simulink model "nmsRR"  (R2021a)
settings: Solver=ode15s  StartTime=0.0  StopTime=t  MaxStep=1e-2  RelTol=1e-2
StartFcn:
  | tic
StopFcn:
  | toc
  | 
  | 
  | %if GimbalLockFlag
  |  % fprintf(2, 'Almost reached Gimbal Lock of IMU. Simulation stopped.\n')
  | %end
  | 
  | %fprintf('Elapsed time: %4.2f sec (%4.2f%% realtime)\n', a, tout(end)/a*100)
undefined symbols (not defined in the file): Balance02, Balance13, BalanceTrunk, BasisStim, CompensateSwing, CompliantLeg, FlexAnkle, Ground, ICs, init_des_left, init_des_right, init_l_left, init_l_right, init_q_del, init_sensor_body, init_sensor_world, init_v_left, init_v_right, LateralControl, mParams, PreventKneeOverextension, StepDur, Target02, Target13, theta0, X, Y, Z
libraries: simulink_extras x133, nesl_utility x105, sm_lib x88, simulink x72, robotcorelib x5, dspinverses x5, dspswit3 x2, vrlib x2, robotmaniplib x1
(part 4 of 8)

== system nmsRR/Body and Contact Model/L Leg/Thigh ==
  Solid : sm_lib/Body Elements/Brick Solid  Commented=on  GraphicAmbientColor=[0.15 0.15 0.15 1.0]  BasedOnType=Density  BrickDimensions="[mParams.bodies.thigh.d  mParams.bodies.thigh.l*(1-mParams.bodies.thigh.ThPos)   mParams.bodies.thigh.b]"  BrickDimensionUnits=m  CenterOfMass=-mParams.bodies.thigh.CG*(1-mParams.bodies.thigh.ThPos)  CenterOfMassUnits=m  GraphicDiffuseColor=[1 0.5 0.5]  Density=2.7  DensityUnits=g/cm^3  DoExposeReferenceFrame=on  GraphicEmissiveColor=[0 0 0 1.0]  ExportEntireGeometry=off  SerializedFrames=<Frames/>  MarkerShape=Sphere  MarkerSize=10  GraphicType=FromGeometry  InertiaType=Custom  Mass=mParams.bodies.thigh.m*(1-mParams.bodies.thigh.ThPos)  MassUnits=kg  MomentsOfInertia=mParams.bodies.thigh.In*[(1-mParams.bodies.thigh.ThPos); (1-mParams.bodies.thigh.ThPos)^3; (1-mParams.bodies.thigh.ThPos)^3]  MomentsOfInertiaUnits=kg*m^2  GraphicOpacity=1.0  ProductsOfInertia=[0 0 0]  ProductsOfInertiaUnits=kg*m^2  GraphicShininess=75  GraphicSpecularColor=[0.5 0.5 0.5 1.0]  GraphicVisPropType=SimpleVisualProperties
  Solid1 : sm_lib/Body Elements/Brick Solid  GraphicAmbientColor=[0.15 0.15 0.15 1.0]  BasedOnType=Density  BrickDimensions=[mParams.bodies.thigh.d mParams.bodies.thigh.l mParams.bodies.thigh.b]  BrickDimensionUnits=m  CenterOfMass=mParams.bodies.thigh.CG  CenterOfMassUnits=m  GraphicDiffuseColor=[1 0.5 0.5]  Density=2.7  DensityUnits=g/cm^3  DoExposeReferenceFrame=on  GraphicEmissiveColor=[0 0 0 1.0]  ExportEntireGeometry=off  SerializedFrames=<Frames><Frame><Id>Frame1</Id><Value><Name>F1</Name><Origin><Source>CenterOfMassFrame</Source><FeatureName></FeatureName></Origin><PrimaryAxis><DefinedDirection>+Z</DefinedDirection><Source>ReferenceFrame</Source><SourceDirection>+Z</SourceDirection><FeatureName></FeatureName></PrimaryAxis><SecondaryAxis><DefinedDirection>+X</DefinedDirection><Source>ReferenceFrame</Source><SourceDirection>+X</SourceDirection><FeatureName></FeatureName></SecondaryAxis></Value></Frame></Frames>  MarkerShape=Sphere  MarkerSize=10  GraphicType=FromGeometry  InertiaType=Custom  Mass=mParams.bodies.thigh.m  MassUnits=kg  MomentsOfInertia=mParams.bodies.thigh.In  MomentsOfInertiaUnits=kg*m^2  GraphicOpacity=1.0  ProductsOfInertia=[0 0 0]  ProductsOfInertiaUnits=kg*m^2  GraphicShininess=75  GraphicSpecularColor=[0.5 0.5 0.5 1.0]  GraphicVisPropType=SimpleVisualProperties
  Transform CG to MidSegment : sm_lib/Frames and Transforms/Rigid Transform  TranslationMethod=Cartesian  TranslationStandardOffset=0  TranslationLengthUnit=m  TranslationStandardAxis=+Y  TranslationCartesianOffset=[0 -mParams.bodies.thigh.l/2 0]  TranslationROffset=0  TranslationROffsetUnits=m  TranslationZOffset=0  TranslationZOffsetUnits=m  TranslationThetaOffset=0  TranslationThetaOffsetUnits=deg  RotationMethod=None  RotationAngleUnits=deg  RotationStandardAxis=+X  RotationAngle=90  RotationArbitraryAxis=[0 0 1]  FollAlignAxisA=+X  BaseAlignAxisA=+Y  FollAlignAxisB=+Y  BaseAlignAxisB=+Z  RotationSequenceAxes=FollowerAxes  RotationSequence=XYX  RotationSequenceAngles=[0 0 0]  RotationSequenceAnglesUnits=deg  RotationMatrix=[1 0 0; 0 1 0; 0 0 1]
  Transform CS1 to MidSegment : sm_lib/Frames and Transforms/Rigid Transform  TranslationMethod=Cartesian  TranslationStandardOffset=0  TranslationLengthUnit=m  TranslationStandardAxis=+Y  TranslationCartesianOffset=[0 -mParams.bodies.thigh.l/2 0]  TranslationROffset=0  TranslationROffsetUnits=m  TranslationZOffset=0  TranslationZOffsetUnits=m  TranslationThetaOffset=0  TranslationThetaOffsetUnits=deg  RotationMethod=None  RotationAngleUnits=deg  RotationStandardAxis=+X  RotationAngle=-90  RotationArbitraryAxis=[0 0 1]  FollAlignAxisA=+X  BaseAlignAxisA=+Y  FollAlignAxisB=+Y  BaseAlignAxisB=+Z  RotationSequenceAxes=FollowerAxes  RotationSequence=XYX  RotationSequenceAngles=[0 0 0]  RotationSequenceAnglesUnits=deg  RotationMatrix=[1 0 0; 0 1 0; 0 0 1]
  CS1 : PMIOPort  Side=Left
  CS2 : PMIOPort  Port=2  Side=Right
  connections:
  Transform CG to MidSegment/LConn1 -- Solid1/RConn1 -- Transform CS1 to MidSegment/RConn1
  Transform CS1 to MidSegment/LConn1 -- CS1/RConn1
  Transform CG to MidSegment/RConn1 -- CS2/RConn1

== system nmsRR/Body and Contact Model/Push in x-direction/ Timer Phase 1 ==
  R : Inport
  Clock1 : Clock
  Clock3 : Clock
      settings: Decimation=4
  NOT : Logic  Operator=NOT  AllPortsSameDT=off  OutDataTypeStr=boolean
  Resettable Subsystem : Subsystem  TreatAsAtomicUnit=on
  Sum1 : Sum  Inputs=|+-  InputSameDT=on  SaturateOnIntegerOverflow=on  OutDataTypeStr=Inherit: Same as first input
  Switch2 : Switch  Criteria=u2 > Threshold  RndMeth=Zero  ZeroCross=off
  Out : Outport  VectorParamsAs1DForOutWhenUnconnected=off
  wires:
  Clock1/1 -> Sum1/1
  Clock3/1 -> Switch2/3, Resettable Subsystem/1(In1)
  Sum1/1 -> Out/1
  R/1 -> NOT/1, Switch2/2
  Switch2/1 -> Sum1/2
  Resettable Subsystem/1(Out1) -> Switch2/1
  NOT/1 -> Resettable Subsystem/Enable

== system nmsRR/Body and Contact Model/Push in y-direction/ Timer Phase 1 ==
  R : Inport
  Clock1 : Clock
  Clock3 : Clock
      settings: Decimation=4
  NOT : Logic  Operator=NOT  AllPortsSameDT=off  OutDataTypeStr=boolean
  Resettable Subsystem : Subsystem  TreatAsAtomicUnit=on
  Sum1 : Sum  Inputs=|+-  InputSameDT=on  SaturateOnIntegerOverflow=on  OutDataTypeStr=Inherit: Same as first input
  Switch2 : Switch  Criteria=u2 > Threshold  RndMeth=Zero  ZeroCross=off
  Out : Outport  VectorParamsAs1DForOutWhenUnconnected=off
  wires:
  Clock1/1 -> Sum1/1
  Clock3/1 -> Switch2/3, Resettable Subsystem/1(In1)
  Sum1/1 -> Out/1
  R/1 -> NOT/1, Switch2/2
  Switch2/1 -> Sum1/2
  Resettable Subsystem/1(Out1) -> Switch2/1
  NOT/1 -> Resettable Subsystem/Enable

== system nmsRR/Body and Contact Model/R Leg/Ankle Mechanical Limits ==
  note: Overflexion Torque
  note: Joint Limits
  note: Overextension Torque
  dq [rad/s] : Inport
  q [rad] : Inport  Port=2
  Gain1 : Gain  Gain=mParams.joints.ankle.kStop
  Gain2 : Gain  Gain=-1
  Gain3 : Gain  Gain=mParams.joints.ankle.kStop
  Gain4 : Gain  Gain=1/mParams.joints.ankle.wMaxStop
  Gain5 : Gain  Gain=-1
  Gain6 : Gain  Gain=-1
  Limit Knee Range : simulink/Logic and Bit Operations/Interval Test  Commented=on  IntervalClosedRight=on  uplimit=mParams.joints.ankle.MaxPitch + 20*pi/180  IntervalClosedLeft=on  lowlimit=mParams.joints.ankle.MinPitch - 20*pi/180  OutDataTypeStr=boolean
      settings: AttributesFormatString=|
      | Lower limits: %<lowlimit>
      | Upper limits: %<uplimit>
  Logical Operator3 : Logic  Commented=on  Operator=NOT  AllPortsSameDT=off  OutDataTypeStr=boolean
  Product1 : Product  Inputs=4
  Product2 : Product  Inputs=4
  Stop Simulation1 : Stop  Commented=on
  Sum : Sum  Inputs=|+-
  Sum1 : Sum  Inputs=|+-
  Sum2 : Sum
  Sum3 : Sum  Inputs=|-+
  Sum4 : Sum  Inputs=|-+
  above upper limit? : simulink/Logic and Bit Operations/Compare To Zero  relop=>  OutDataTypeStr=boolean  ZeroCross=off
  below lower limit? : simulink/Logic and Bit Operations/Compare To Zero  relop=<  OutDataTypeStr=boolean  ZeroCross=off
  const : Constant
  const1 : Constant
  mech limit pushes back? : simulink/Logic and Bit Operations/Compare To Zero  relop=>  OutDataTypeStr=boolean  ZeroCross=off
  mech limit pushes back?. : simulink/Logic and Bit Operations/Compare To Zero  relop=>  OutDataTypeStr=boolean  ZeroCross=off
  overextension angle : Constant  Value=mParams.joints.ankle.MaxPitch
  overflexion angle : Constant  Value=mParams.joints.ankle.MinPitch
  tau [Nm] : Outport  VectorParamsAs1DForOutWhenUnconnected=off
  wires:
  Gain5/1 -> Sum2/2
  Gain4/1 -> Gain2/1, Sum4/1
  const1/1 -> Sum4/2
  Sum4/1 -> Product2/3, mech limit pushes back?./1
  Gain1/1 -> Product2/2, below lower limit?/1
  mech limit pushes back?./1 -> Product2/4
  below lower limit?/1 -> Product2/1
  Product2/1 -> Gain5/1
  Product1/1 -> Gain6/1
  above upper limit?/1 -> Product1/1
  mech limit pushes back?/1 -> Product1/4
  Gain3/1 -> above upper limit?/1, Product1/2
  Sum3/1 -> mech limit pushes back?/1, Product1/3
  const/1 -> Sum3/2
  dq [rad/s]/1 -> Gain4/1
  overextension angle/1 -> Sum/2
  q [rad]/1 -> Sum/1, Limit Knee Range/1, Sum1/1
  Sum/1 -> Gain3/1
  Sum1/1 -> Gain1/1
  overflexion angle/1 -> Sum1/2
  Sum2/1 -> tau [Nm]/1
  Gain2/1 -> Sum3/1
  Gain6/1 -> Sum2/1
  Limit Knee Range/1 -> Logical Operator3/1
  Logical Operator3/1 -> Stop Simulation1/1

== system nmsRR/Body and Contact Model/R Leg/Foot1 ==
  "  XYZ Sensor " : Subsystem
  "  XYZ Sensor Ball left" : Subsystem
  B Transform : sm_lib/Frames and Transforms/Rigid Transform  TranslationMethod=Cartesian  TranslationStandardOffset=0  TranslationLengthUnit=m  TranslationStandardAxis=+Y  TranslationCartesianOffset=[ mParams.bodies.foot.compensation mParams.bodies.foot.l/2 0]  TranslationROffset=0  TranslationROffsetUnits=m  TranslationZOffset=0  TranslationZOffsetUnits=m  TranslationThetaOffset=0  TranslationThetaOffsetUnits=deg  RotationMethod=None  RotationAngleUnits=deg  RotationStandardAxis=+X  RotationAngle=90  RotationArbitraryAxis=[0 0 1]  FollAlignAxisA=+X  BaseAlignAxisA=+Y  FollAlignAxisB=+Y  BaseAlignAxisB=+Z  RotationSequenceAxes=FollowerAxes  RotationSequence=XYX  RotationSequenceAngles=[0 0 0]  RotationSequenceAnglesUnits=deg  RotationMatrix=[1 0 0; 0 1 0; 0 0 1]
  LB Transform : sm_lib/Frames and Transforms/Rigid Transform  TranslationMethod=Cartesian  TranslationStandardOffset=0  TranslationLengthUnit=m  TranslationStandardAxis=+Y  TranslationCartesianOffset="[mParams.bodies.foot.l/2 -mParams.bodies.foot.compensation  -mParams.bodies.foot.BallWidth/2]"  TranslationROffset=0  TranslationROffsetUnits=m  TranslationZOffset=0  TranslationZOffsetUnits=m  TranslationThetaOffset=0  TranslationThetaOffsetUnits=deg  RotationMethod=None  RotationAngleUnits=deg  RotationStandardAxis=+X  RotationAngle=90  RotationArbitraryAxis=[0 0 1]  FollAlignAxisA=+X  BaseAlignAxisA=+Y  FollAlignAxisB=+Y  BaseAlignAxisB=+Z  RotationSequenceAxes=FollowerAxes  RotationSequence=XYX  RotationSequenceAngles=[0 0 0]  RotationSequenceAnglesUnits=deg  RotationMatrix=[1 0 0; 0 1 0; 0 0 1]
  LH Transform : sm_lib/Frames and Transforms/Rigid Transform  TranslationMethod=Cartesian  TranslationStandardOffset=0  TranslationLengthUnit=m  TranslationStandardAxis=+Y  TranslationCartesianOffset="[-mParams.bodies.foot.l/2 -mParams.bodies.foot.compensation  -mParams.bodies.foot.HeelWidth/2]"  TranslationROffset=0  TranslationROffsetUnits=m  TranslationZOffset=0  TranslationZOffsetUnits=m  TranslationThetaOffset=0  TranslationThetaOffsetUnits=deg  RotationMethod=None  RotationAngleUnits=deg  RotationStandardAxis=+X  RotationAngle=90  RotationArbitraryAxis=[0 0 1]  FollAlignAxisA=+X  BaseAlignAxisA=+Y  FollAlignAxisB=+Y  BaseAlignAxisB=+Z  RotationSequenceAxes=FollowerAxes  RotationSequence=XYX  RotationSequenceAngles=[0 0 0]  RotationSequenceAnglesUnits=deg  RotationMatrix=[1 0 0; 0 1 0; 0 0 1]
  RB Transform : sm_lib/Frames and Transforms/Rigid Transform  TranslationMethod=Cartesian  TranslationStandardOffset=0  TranslationLengthUnit=m  TranslationStandardAxis=+Z  TranslationCartesianOffset="[mParams.bodies.foot.l/2 -mParams.bodies.foot.compensation  mParams.bodies.foot.BallWidth/2]"  TranslationROffset=0  TranslationROffsetUnits=m  TranslationZOffset=0  TranslationZOffsetUnits=m  TranslationThetaOffset=0  TranslationThetaOffsetUnits=deg  RotationMethod=None  RotationAngleUnits=deg  RotationStandardAxis=+Z  RotationAngle=0.0  RotationArbitraryAxis=[0 0 1]  FollAlignAxisA=+X  BaseAlignAxisA=+Y  FollAlignAxisB=+Y  BaseAlignAxisB=+Z  RotationSequenceAxes=FollowerAxes  RotationSequence=XYX  RotationSequenceAngles=[0 0 0]  RotationSequenceAnglesUnits=deg  RotationMatrix=[1 0 0; 0 1 0; 0 0 1]
  RH Transform : sm_lib/Frames and Transforms/Rigid Transform  TranslationMethod=Cartesian  TranslationStandardOffset=0  TranslationLengthUnit=m  TranslationStandardAxis=+Z  TranslationCartesianOffset="[-mParams.bodies.foot.l/2 -mParams.bodies.foot.compensation  mParams.bodies.foot.HeelWidth/2]"  TranslationROffset=0  TranslationROffsetUnits=m  TranslationZOffset=0  TranslationZOffsetUnits=m  TranslationThetaOffset=0  TranslationThetaOffsetUnits=deg  RotationMethod=None  RotationAngleUnits=deg  RotationStandardAxis=+Z  RotationAngle=0.0  RotationArbitraryAxis=[0 0 1]  FollAlignAxisA=+X  BaseAlignAxisA=+Y  FollAlignAxisB=+Y  BaseAlignAxisB=+Z  RotationSequenceAxes=FollowerAxes  RotationSequence=XYX  RotationSequenceAngles=[0 0 0]  RotationSequenceAnglesUnits=deg  RotationMatrix=[1 0 0; 0 1 0; 0 0 1]
  Solid1 : sm_lib/Body Elements/Brick Solid  GraphicAmbientColor=[0.15 0.15 0.15 1.0]  BasedOnType=Density  BrickDimensions="[mParams.bodies.foot.l  mParams.bodies.foot.d mParams.bodies.foot.b]"  BrickDimensionUnits=m  CenterOfMass=mParams.bodies.foot.CG  CenterOfMassUnits=m  GraphicDiffuseColor=[1 0.5 0.5]  Density=2.7  DensityUnits=g/cm^3  DoExposeReferenceFrame=on  GraphicEmissiveColor=[0 0 0 1.0]  ExportEntireGeometry=off  SerializedFrames=<Frames><Frame><Id>Frame1</Id><Value><Name>CG</Name><Origin><Source>CenterOfMassFrame</Source><FeatureName></FeatureName></Origin><PrimaryAxis><DefinedDirection>+Z</DefinedDirection><Source>ReferenceFrame</Source><SourceDirection>+Z</SourceDirection><FeatureName></FeatureName></PrimaryAxis><SecondaryAxis><DefinedDirection>+X</DefinedDirection><Source>ReferenceFrame</Source><SourceDirection>+X</SourceDirection><FeatureName></FeatureName></SecondaryAxis></Value></Frame></Frames>  MarkerShape=Sphere  MarkerSize=10  GraphicType=FromGeometry  InertiaType=Custom  Mass=mParams.bodies.foot.m  MassUnits=kg  MomentsOfInertia=mParams.bodies.foot.In  MomentsOfInertiaUnits=kg*m^2  GraphicOpacity=1.0  ProductsOfInertia=[0 0 0]  ProductsOfInertiaUnits=kg*m^2  GraphicShininess=75  GraphicSpecularColor=[0.5 0.5 0.5 1.0]  GraphicVisPropType=SimpleVisualProperties
  Terminator : Terminator
  Terminator1 : Terminator
  To Workspace4 : ToWorkspace  VariableName=Ball_right  SampleTime=-1
      settings: Save2DSignal=2-D array (concatenate along first dimension)
  Transform Ankle to MidSegment : sm_lib/Frames and Transforms/Rigid Transform  TranslationMethod=Cartesian  TranslationStandardOffset=0  TranslationLengthUnit=m  TranslationStandardAxis=+Y  TranslationCartesianOffset=mParams.bodies.foot.AnkleToMid  TranslationROffset=0  TranslationROffsetUnits=m  TranslationZOffset=0  TranslationZOffsetUnits=m  TranslationThetaOffset=0  TranslationThetaOffsetUnits=deg  RotationMethod=RotationSequence  RotationAngleUnits=deg  RotationStandardAxis=+X  RotationAngle=-90  RotationArbitraryAxis=[0 0 1]  FollAlignAxisA=+X  BaseAlignAxisA=+Y  FollAlignAxisB=+Y  BaseAlignAxisB=+Z  RotationSequenceAxes=FollowerAxes  RotationSequence=ZXY  RotationSequenceAngles=[90 0 0]  RotationSequenceAnglesUnits=deg  RotationMatrix=[1 0 0; 0 1 0; 0 0 1]
  CS1 : PMIOPort  Side=Left
  Left Ball : PMIOPort  Port=2  Side=Right
  Left Heel : PMIOPort  Port=3  Side=Left
  Right Ball : PMIOPort  Port=4  Side=Right
  Right Heel : PMIOPort  Port=5  Side=Left
  Out1 : Outport  VectorParamsAs1DForOutWhenUnconnected=off
  tag scope: Ball_right=global
  wires:
  "  XYZ Sensor "/1(p_bLH [m x3]) -> Out1/1
  "  XYZ Sensor Ball left"/2(v_bLH [m/s x3]) -> Terminator/1
  "  XYZ Sensor Ball left"/1(p_bLH [m x3]) -> To Workspace4/1, [Ball_right]
  "  XYZ Sensor "/2(v_bLH [m/s x3]) -> Terminator1/1
  connections:
  Transform Ankle to MidSegment/RConn1 -- B Transform/LConn1 -- RB Transform/LConn1 -- Solid1/RConn1 -- RH Transform/LConn1 -- LH Transform/LConn1 -- LB Transform/LConn1
  Transform Ankle to MidSegment/LConn1 -- CS1/RConn1
  Left Heel/RConn1 -- LH Transform/RConn1
  Left Ball/RConn1 -- LB Transform/RConn1
  Right Heel/RConn1 -- RH Transform/RConn1
  Right Ball/RConn1 -- RB Transform/RConn1
  Solid1/LConn1 -- "  XYZ Sensor "/LConn1
  B Transform/RConn1 -- "  XYZ Sensor Ball left"/LConn1

== system nmsRR/Body and Contact Model/R Leg/Hip Pitch Mechanical Limits ==
  note: Overextension Torque
  note: Joint Limits
  note: Overflexion Torque
  dq [rad/s] : Inport
  q [rad] : Inport  Port=2
  Gain1 : Gain  Gain=mParams.joints.hip.kStop
  Gain2 : Gain  Gain=-1
  Gain3 : Gain  Gain=mParams.joints.hip.kStop
  Gain4 : Gain  Gain=1/mParams.joints.hip.wMaxStop
  Gain5 : Gain  Gain=-1
  Gain6 : Gain  Gain=-1
  Limit Joint Range : simulink/Logic and Bit Operations/Interval Test  Commented=on  IntervalClosedRight=on  uplimit=mParams.joints.hip.MaxPitch + 20*pi/180  IntervalClosedLeft=on  lowlimit=mParams.joints.hip.MinPitch - 20*pi/180  OutDataTypeStr=boolean
      settings: AttributesFormatString=|
      | Lower limits: %<lowlimit>
      | Upper limits: %<uplimit>
  Logical Operator3 : Logic  Commented=on  Operator=NOT  AllPortsSameDT=off  OutDataTypeStr=boolean
  Product1 : Product  Inputs=4
  Product2 : Product  Inputs=4
  Stop Simulation1 : Stop  Commented=on
  Sum : Sum  Inputs=|+-
  Sum1 : Sum  Inputs=|+-
  Sum2 : Sum
  Sum3 : Sum  Inputs=|-+
  Sum4 : Sum  Inputs=|-+
  above upper limit? : simulink/Logic and Bit Operations/Compare To Zero  relop=>  OutDataTypeStr=boolean  ZeroCross=off
  below lower limit? : simulink/Logic and Bit Operations/Compare To Zero  relop=<  OutDataTypeStr=boolean  ZeroCross=off
  const : Constant
  const1 : Constant
  mech limit pushes back? : simulink/Logic and Bit Operations/Compare To Zero  relop=>  OutDataTypeStr=boolean  ZeroCross=off
  mech limit pushes back?. : simulink/Logic and Bit Operations/Compare To Zero  relop=>  OutDataTypeStr=boolean  ZeroCross=off
  overextension angle : Constant  Value=mParams.joints.hip.MaxPitch
  overflexion angle : Constant  Value=mParams.joints.hip.MinPitch
  tau [Nm] : Outport  VectorParamsAs1DForOutWhenUnconnected=off
  wires:
  Logical Operator3/1 -> Stop Simulation1/1
  Limit Joint Range/1 -> Logical Operator3/1
  Gain6/1 -> Sum2/1
  Gain2/1 -> Sum3/1
  Sum2/1 -> tau [Nm]/1
  overflexion angle/1 -> Sum1/2
  Sum1/1 -> Gain1/1
  Sum/1 -> Gain3/1
  q [rad]/1 -> Sum/1, Sum1/1, Limit Joint Range/1
  overextension angle/1 -> Sum/2
  dq [rad/s]/1 -> Gain4/1
  const/1 -> Sum3/2
  Sum3/1 -> Product1/3, mech limit pushes back?/1
  Gain3/1 -> Product1/2, above upper limit?/1
  mech limit pushes back?/1 -> Product1/4
  above upper limit?/1 -> Product1/1
  Product1/1 -> Gain6/1
  Product2/1 -> Gain5/1
  below lower limit?/1 -> Product2/1
  mech limit pushes back?./1 -> Product2/4
  Gain1/1 -> Product2/2, below lower limit?/1
  Sum4/1 -> mech limit pushes back?./1, Product2/3
  const1/1 -> Sum4/2
  Gain4/1 -> Sum4/1, Gain2/1
  Gain5/1 -> Sum2/2

== system nmsRR/Body and Contact Model/R Leg/Hip Roll Mechanical Limits ==
  note: Overextension Torque
  note: Joint Limits
  note: Overflexion Torque
  dq [rad/s] : Inport
  q [rad] : Inport  Port=2
  Gain1 : Gain  Gain=mParams.joints.hip.kStop
  Gain2 : Gain  Gain=-1
  Gain3 : Gain  Gain=mParams.joints.hip.kStop
  Gain4 : Gain  Gain=1/mParams.joints.hip.wMaxStop
  Gain5 : Gain  Gain=-1
  Gain6 : Gain  Gain=-1
  Limit Joint Range : simulink/Logic and Bit Operations/Interval Test  Commented=on  IntervalClosedRight=on  uplimit=mParams.joints.hip.MaxRoll + 20*pi/180  IntervalClosedLeft=on  lowlimit=mParams.joints.hip.MinRoll - 20*pi/180  OutDataTypeStr=boolean
      settings: AttributesFormatString=|
      | Lower limits: %<lowlimit>
      | Upper limits: %<uplimit>
  Logical Operator3 : Logic  Commented=on  Operator=NOT  AllPortsSameDT=off  OutDataTypeStr=boolean
  Product1 : Product  Inputs=4
  Product2 : Product  Inputs=4
  Stop Simulation1 : Stop  Commented=on
  Sum : Sum  Inputs=|+-
  Sum1 : Sum  Inputs=|+-
  Sum2 : Sum
  Sum3 : Sum  Inputs=|-+
  Sum4 : Sum  Inputs=|-+
  above upper limit? : simulink/Logic and Bit Operations/Compare To Zero  relop=>  OutDataTypeStr=boolean  ZeroCross=off
  below lower limit? : simulink/Logic and Bit Operations/Compare To Zero  relop=<  OutDataTypeStr=boolean  ZeroCross=off
  const : Constant
  const1 : Constant
  mech limit pushes back? : simulink/Logic and Bit Operations/Compare To Zero  relop=>  OutDataTypeStr=boolean  ZeroCross=off
  mech limit pushes back?. : simulink/Logic and Bit Operations/Compare To Zero  relop=>  OutDataTypeStr=boolean  ZeroCross=off
  overextension angle : Constant  Value=mParams.joints.hip.MaxRoll
  overflexion angle : Constant  Value=mParams.joints.hip.MinRoll
  tau [Nm] : Outport  VectorParamsAs1DForOutWhenUnconnected=off
  wires:
  Limit Joint Range/1 -> Logical Operator3/1
  Gain6/1 -> Sum2/1
  Gain2/1 -> Sum3/1
  Sum2/1 -> tau [Nm]/1
  overflexion angle/1 -> Sum1/2
  Sum1/1 -> Gain1/1
  Sum/1 -> Gain3/1
  q [rad]/1 -> Sum/1, Sum1/1, Limit Joint Range/1
  overextension angle/1 -> Sum/2
  dq [rad/s]/1 -> Gain4/1
  const/1 -> Sum3/2
  Sum3/1 -> Product1/3, mech limit pushes back?/1
  Gain3/1 -> Product1/2, above upper limit?/1
  mech limit pushes back?/1 -> Product1/4
  above upper limit?/1 -> Product1/1
  Product1/1 -> Gain6/1
  Product2/1 -> Gain5/1
  below lower limit?/1 -> Product2/1
  mech limit pushes back?./1 -> Product2/4
  Gain1/1 -> Product2/2, below lower limit?/1
  Sum4/1 -> mech limit pushes back?./1, Product2/3
  const1/1 -> Sum4/2
  Gain4/1 -> Sum4/1, Gain2/1
  Gain5/1 -> Sum2/2
  Logical Operator3/1 -> Stop Simulation1/1

== system nmsRR/Body and Contact Model/R Leg/Knee Mechanical Limits ==
  note: Overextension Torque
  note: Joint Limits
  note: Overflexion Torque
  dq [rad/s] : Inport
  q [rad] : Inport  Port=2
  Gain1 : Gain  Gain=mParams.joints.knee.kStop
  Gain2 : Gain  Gain=-1
  Gain3 : Gain  Gain=mParams.joints.knee.kStop
  Gain4 : Gain  Gain=1/mParams.joints.knee.wMaxStop
  Gain5 : Gain  Gain=-1
  Gain6 : Gain  Gain=-1
  Limit Knee Range : simulink/Logic and Bit Operations/Interval Test  IntervalClosedRight=on  uplimit=mParams.joints.knee.MaxPitch + 20*pi/180  IntervalClosedLeft=on  lowlimit=mParams.joints.knee.MinPitch - 20*pi/180  OutDataTypeStr=boolean
      settings: AttributesFormatString=|
      | Lower limits: %<lowlimit>
      | Upper limits: %<uplimit>
  Logical Operator3 : Logic  Operator=NOT  AllPortsSameDT=off  OutDataTypeStr=boolean
  Product1 : Product  Inputs=4
  Product2 : Product  Inputs=4
  Stop Simulation1 : Stop
  Sum : Sum  Inputs=|+-
  Sum1 : Sum  Inputs=|+-
  Sum2 : Sum
  Sum3 : Sum  Inputs=|-+
  Sum4 : Sum  Inputs=|-+
  above upper limit? : simulink/Logic and Bit Operations/Compare To Zero  relop=>  OutDataTypeStr=boolean  ZeroCross=off
  below lower limit? : simulink/Logic and Bit Operations/Compare To Zero  relop=<  OutDataTypeStr=boolean  ZeroCross=off
  const : Constant
  const1 : Constant
  mech limit pushes back? : simulink/Logic and Bit Operations/Compare To Zero  relop=>  OutDataTypeStr=boolean  ZeroCross=off
  mech limit pushes back?. : simulink/Logic and Bit Operations/Compare To Zero  relop=>  OutDataTypeStr=boolean  ZeroCross=off
  overextension angle : Constant  Value=mParams.joints.knee.MaxPitch
  overflexion angle : Constant  Value=mParams.joints.knee.MinPitch
  tau [Nm] : Outport  VectorParamsAs1DForOutWhenUnconnected=off
  wires:
  Logical Operator3/1 -> Stop Simulation1/1
  Limit Knee Range/1 -> Logical Operator3/1
  Gain6/1 -> Sum2/1
  Gain2/1 -> Sum3/1
  Sum2/1 -> tau [Nm]/1
  overflexion angle/1 -> Sum1/2
  Sum1/1 -> Gain1/1
  Sum/1 -> Gain3/1
  q [rad]/1 -> Sum1/1, Limit Knee Range/1, Sum/1
  overextension angle/1 -> Sum/2
  dq [rad/s]/1 -> Gain4/1
  const/1 -> Sum3/2
  Sum3/1 -> Product1/3, mech limit pushes back?/1
  Gain3/1 -> Product1/2, above upper limit?/1
  mech limit pushes back?/1 -> Product1/4
  above upper limit?/1 -> Product1/1
  Product1/1 -> Gain6/1
  Product2/1 -> Gain5/1
  below lower limit?/1 -> Product2/1
  mech limit pushes back?./1 -> Product2/4
  Gain1/1 -> below lower limit?/1, Product2/2
  Sum4/1 -> mech limit pushes back?./1, Product2/3
  const1/1 -> Sum4/2
  Gain4/1 -> Sum4/1, Gain2/1
  Gain5/1 -> Sum2/2

== system nmsRR/Body and Contact Model/R Leg/Rotation Sensor Knee ==
  note: Rotation Sensor in World Frame
  Coordinate Transformation Conversion1 : robotcorelib/Coordinate Transformation Conversion  InputRepresentation=Quaternion  InputEulerSequence=ZYX  ShowTrVecInputPort=on  OutputRepresentation=Euler Angles  OutputEulerSequence=XYZ  ShowTrVecOutputPort=on  SimulateUsing=Code generation
      settings: SourceProductBaseCode=NV,RO,RR,UV
  Coordinate Transformation Conversion2 : robotcorelib/Coordinate Transformation Conversion  InputRepresentation=Quaternion  InputEulerSequence=ZYX  ShowTrVecInputPort=on  OutputRepresentation=Rotation Matrix  OutputEulerSequence=XYZ  ShowTrVecOutputPort=on  SimulateUsing=Code generation
      settings: SourceProductBaseCode=NV,RO,RR,UV
  Frame Sensor : sm_lib/Frames and Transforms/Transform Sensor  MeasurementFrame=World  SenseAngle=off  SenseAxis=off  SenseAngle1=off  SenseAngle2=off  SenseAngle3=off  SenseQ=on  SenseR=off  SenseOmegaX=off  SenseOmegaY=off  SenseOmegaZ=off  SenseOmega1=off  SenseOmega2=off  SenseOmega3=off  SenseQDot=off  SenseRDot=off  SenseAlphaX=off  SenseAlphaY=off  SenseAlphaZ=off  SenseAlpha1=off  SenseAlpha2=off  SenseAlpha3=off  SenseQDDot=off  SenseRDDot=off  SenseX=off  SenseY=off  SenseZ=off  SenseRad=off  SenseAzim=off  SenseDist=off  SenseInc=off  SenseXDot=off  SenseYDot=off  SenseZDot=off  SenseRadDot=off  SenseAzimDot=off  SenseDistDot=off  SenseIncDot=off  SenseXDDot=off  SenseYDDot=off  SenseZDDot=off  SenseRadDDot=off  SenseAzimDDot=off  SenseDistDDot=off  SenseIncDDot=off
  PS-Simulink Converter12 : nesl_utility/PS-Simulink Converter  PhysicalDomain=network_engine_domain  SubClassName=ps_output  LeftPortType=input  RightPortType=output  PseudoPeriodic=off  Frequencies=[]  Unit=1  AffineConversion=off
      settings: SourceProductBaseCode=PW,SS
  World Frame : sm_lib/Frames and Transforms/World Frame
  frame : PMIOPort  Side=Left
  rotation [rad] : Outport  VectorParamsAs1DForOutWhenUnconnected=off
  Rotation Matrix : Outport  Port=2  VectorParamsAs1DForOutWhenUnconnected=off
  wires:
  PS-Simulink Converter12/1 -> Coordinate Transformation Conversion2/1, Coordinate Transformation Conversion1/1
  Coordinate Transformation Conversion1/1 -> rotation [rad]/1
  Coordinate Transformation Conversion2/1 -> Rotation Matrix/1
  connections:
  Frame Sensor/RConn1 -- frame/RConn1
  World Frame/RConn1 -- Frame Sensor/LConn1
  PS-Simulink Converter12/LConn1 -- Frame Sensor/RConn2

== system nmsRR/Body and Contact Model/R Leg/Sensor Right Ankle ==
  note: Position and Velocity Sensor in World Frame
  Frame Sensor : sm_lib/Frames and Transforms/Transform Sensor  MeasurementFrame=Base  SenseAngle=off  SenseAxis=off  SenseAngle1=off  SenseAngle2=off  SenseAngle3=off  SenseQ=off  SenseR=off  SenseOmegaX=off  SenseOmegaY=off  SenseOmegaZ=off  SenseOmega1=off  SenseOmega2=off  SenseOmega3=off  SenseQDot=off  SenseRDot=off  SenseAlphaX=off  SenseAlphaY=off  SenseAlphaZ=off  SenseAlpha1=off  SenseAlpha2=off  SenseAlpha3=off  SenseQDDot=off  SenseRDDot=off  SenseX=on  SenseY=on  SenseZ=on  SenseRad=off  SenseAzim=off  SenseDist=off  SenseInc=off  SenseXDot=on  SenseYDot=on  SenseZDot=on  SenseRadDot=off  SenseAzimDot=off  SenseDistDot=off  SenseIncDot=off  SenseXDDot=off  SenseYDDot=off  SenseZDDot=off  SenseRadDDot=off  SenseAzimDDot=off  SenseDistDDot=off  SenseIncDDot=off
  Mux : Mux  Inputs=3
  Mux1 : Mux  Inputs=3
  PS-Simulink Converter1 : nesl_utility/PS-Simulink Converter  PhysicalDomain=network_engine_domain  SubClassName=ps_output  LeftPortType=input  RightPortType=output  PseudoPeriodic=off  Frequencies=[]  Unit=m  AffineConversion=off
      settings: SourceProductBaseCode=PW,SS
  PS-Simulink Converter12 : nesl_utility/PS-Simulink Converter  PhysicalDomain=network_engine_domain  SubClassName=ps_output  LeftPortType=input  RightPortType=output  PseudoPeriodic=off  Frequencies=[]  Unit=m  AffineConversion=off
      settings: SourceProductBaseCode=PW,SS
  PS-Simulink Converter2 : nesl_utility/PS-Simulink Converter  PhysicalDomain=network_engine_domain  SubClassName=ps_output  LeftPortType=input  RightPortType=output  PseudoPeriodic=off  Frequencies=[]  Unit=m  AffineConversion=off
      settings: SourceProductBaseCode=PW,SS
  PS-Simulink Converter3 : nesl_utility/PS-Simulink Converter  PhysicalDomain=network_engine_domain  SubClassName=ps_output  LeftPortType=input  RightPortType=output  PseudoPeriodic=off  Frequencies=[]  Unit=m/s  AffineConversion=off
      settings: SourceProductBaseCode=PW,SS
  PS-Simulink Converter4 : nesl_utility/PS-Simulink Converter  PhysicalDomain=network_engine_domain  SubClassName=ps_output  LeftPortType=input  RightPortType=output  PseudoPeriodic=off  Frequencies=[]  Unit=m/s  AffineConversion=off
      settings: SourceProductBaseCode=PW,SS
  PS-Simulink Converter5 : nesl_utility/PS-Simulink Converter  PhysicalDomain=network_engine_domain  SubClassName=ps_output  LeftPortType=input  RightPortType=output  PseudoPeriodic=off  Frequencies=[]  Unit=m/s  AffineConversion=off
      settings: SourceProductBaseCode=PW,SS
  World Frame : sm_lib/Frames and Transforms/World Frame
  Frame : PMIOPort  Side=Left
  Position [m] : Outport  VectorParamsAs1DForOutWhenUnconnected=off
  Velocity [m/s] : Outport  Port=2  VectorParamsAs1DForOutWhenUnconnected=off
  wires:
  PS-Simulink Converter12/1 -> Mux/1
  PS-Simulink Converter1/1 -> Mux/2
  PS-Simulink Converter2/1 -> Mux/3
  Mux/1 -> Position [m]/1
  PS-Simulink Converter5/1 -> Mux1/3
  PS-Simulink Converter4/1 -> Mux1/1
  Mux1/1 -> Velocity [m/s]/1
  PS-Simulink Converter3/1 -> Mux1/2
  connections:
  Frame Sensor/RConn1 -- Frame/RConn1
  PS-Simulink Converter12/LConn1 -- Frame Sensor/RConn2
  Frame Sensor/RConn3 -- PS-Simulink Converter1/LConn1
  Frame Sensor/RConn4 -- PS-Simulink Converter2/LConn1
  Frame Sensor/RConn7 -- PS-Simulink Converter5/LConn1
  Frame Sensor/RConn5 -- PS-Simulink Converter4/LConn1
  Frame Sensor/RConn6 -- PS-Simulink Converter3/LConn1
  World Frame/RConn1 -- Frame Sensor/LConn1

== system nmsRR/Body and Contact Model/R Leg/Shank ==
  Solid : sm_lib/Body Elements/Brick Solid  GraphicAmbientColor=[0.15 0.15 0.15 1.0]  BasedOnType=Density  BrickDimensions="[mParams.bodies.shank.d  mParams.bodies.shank.l mParams.bodies.shank.b]"  BrickDimensionUnits=m  CenterOfMass=mParams.bodies.shank.CG  CenterOfMassUnits=m  GraphicDiffuseColor=[1 0.5 0.5]  Density=2.7  DensityUnits=g/cm^3  DoExposeReferenceFrame=on  GraphicEmissiveColor=[0 0 0 1.0]  ExportEntireGeometry=off  SerializedFrames=<Frames><Frame><Id>Frame1</Id><Value><Name>F1</Name><Origin><Source>CenterOfMassFrame</Source><FeatureName></FeatureName></Origin><PrimaryAxis><DefinedDirection>+Z</DefinedDirection><Source>ReferenceFrame</Source><SourceDirection>+Z</SourceDirection><FeatureName></FeatureName></PrimaryAxis><SecondaryAxis><DefinedDirection>+X</DefinedDirection><Source>ReferenceFrame</Source><SourceDirection>+X</SourceDirection><FeatureName></FeatureName></SecondaryAxis></Value></Frame></Frames>  MarkerShape=Sphere  MarkerSize=10  GraphicType=FromGeometry  InertiaType=Custom  Mass=mParams.bodies.shank.m  MassUnits=kg  MomentsOfInertia=mParams.bodies.shank.In  MomentsOfInertiaUnits=kg*m^2  GraphicOpacity=1.0  ProductsOfInertia=[0 0 0]  ProductsOfInertiaUnits=kg*m^2  GraphicShininess=75  GraphicSpecularColor=[0.5 0.5 0.5 1.0]  GraphicVisPropType=SimpleVisualProperties
  Transform CS1 to MidSegment : sm_lib/Frames and Transforms/Rigid Transform  TranslationMethod=Cartesian  TranslationStandardOffset=0  TranslationLengthUnit=m  TranslationStandardAxis=+Y  TranslationCartesianOffset=[0 -mParams.bodies.shank.l/2 0]  TranslationROffset=0  TranslationROffsetUnits=m  TranslationZOffset=0  TranslationZOffsetUnits=m  TranslationThetaOffset=0  TranslationThetaOffsetUnits=deg  RotationMethod=None  RotationAngleUnits=deg  RotationStandardAxis=+X  RotationAngle=-90  RotationArbitraryAxis=[0 0 1]  FollAlignAxisA=+X  BaseAlignAxisA=+Y  FollAlignAxisB=+Y  BaseAlignAxisB=+Z  RotationSequenceAxes=FollowerAxes  RotationSequence=XYX  RotationSequenceAngles=[0 0 0]  RotationSequenceAnglesUnits=deg  RotationMatrix=[1 0 0; 0 1 0; 0 0 1]
  Transform MidSegment to CS2 : sm_lib/Frames and Transforms/Rigid Transform  TranslationMethod=Cartesian  TranslationStandardOffset=0  TranslationLengthUnit=m  TranslationStandardAxis=+Y  TranslationCartesianOffset=[ 0 -mParams.bodies.shank.l/2 0]  TranslationROffset=0  TranslationROffsetUnits=m  TranslationZOffset=0  TranslationZOffsetUnits=m  TranslationThetaOffset=0  TranslationThetaOffsetUnits=deg  RotationMethod=None  RotationAngleUnits=deg  RotationStandardAxis=+X  RotationAngle=90  RotationArbitraryAxis=[0 0 1]  FollAlignAxisA=+X  BaseAlignAxisA=+Y  FollAlignAxisB=+Y  BaseAlignAxisB=+Z  RotationSequenceAxes=FollowerAxes  RotationSequence=XYX  RotationSequenceAngles=[0 0 0]  RotationSequenceAnglesUnits=deg  RotationMatrix=[1 0 0; 0 1 0; 0 0 1]
  CS1 : PMIOPort  Side=Left
  CS2 : PMIOPort  Port=2  Side=Right
  connections:
  Transform MidSegment to CS2/LConn1 -- Transform CS1 to MidSegment/RConn1 -- Solid/RConn1
  Transform CS1 to MidSegment/LConn1 -- CS1/RConn1
  Transform MidSegment to CS2/RConn1 -- CS2/RConn1

== system nmsRR/Body and Contact Model/R Leg/Thigh ==
  Solid : sm_lib/Body Elements/Brick Solid  Commented=on  GraphicAmbientColor=[0.15 0.15 0.15 1.0]  BasedOnType=Density  BrickDimensions="[mParams.bodies.thigh.d  mParams.bodies.thigh.l*(1-mParams.bodies.thigh.ThPos)   mParams.bodies.thigh.b]"  BrickDimensionUnits=m  CenterOfMass=-mParams.bodies.thigh.CG*(1-mParams.bodies.thigh.ThPos)  CenterOfMassUnits=m  GraphicDiffuseColor=[1 0.5 0.5]  Density=2.7  DensityUnits=g/cm^3  DoExposeReferenceFrame=on  GraphicEmissiveColor=[0 0 0 1.0]  ExportEntireGeometry=off  SerializedFrames=<Frames/>  MarkerShape=Sphere  MarkerSize=10  GraphicType=FromGeometry  InertiaType=Custom  Mass=mParams.bodies.thigh.m*(1-mParams.bodies.thigh.ThPos)  MassUnits=kg  MomentsOfInertia=mParams.bodies.thigh.In*[(1-mParams.bodies.thigh.ThPos); (1-mParams.bodies.thigh.ThPos)^3; (1-mParams.bodies.thigh.ThPos)^3]  MomentsOfInertiaUnits=kg*m^2  GraphicOpacity=1.0  ProductsOfInertia=[0 0 0]  ProductsOfInertiaUnits=kg*m^2  GraphicShininess=75  GraphicSpecularColor=[0.5 0.5 0.5 1.0]  GraphicVisPropType=SimpleVisualProperties
  Solid1 : sm_lib/Body Elements/Brick Solid  GraphicAmbientColor=[0.15 0.15 0.15 1.0]  BasedOnType=Density  BrickDimensions=[mParams.bodies.thigh.d mParams.bodies.thigh.l mParams.bodies.thigh.b]  BrickDimensionUnits=m  CenterOfMass=mParams.bodies.thigh.CG  CenterOfMassUnits=m  GraphicDiffuseColor=[1 0.5 0.5]  Density=2.7  DensityUnits=g/cm^3  DoExposeReferenceFrame=on  GraphicEmissiveColor=[0 0 0 1.0]  ExportEntireGeometry=off  SerializedFrames=<Frames><Frame><Id>Frame1</Id><Value><Name>F1</Name><Origin><Source>CenterOfMassFrame</Source><FeatureName></FeatureName></Origin><PrimaryAxis><DefinedDirection>+Z</DefinedDirection><Source>ReferenceFrame</Source><SourceDirection>+Z</SourceDirection><FeatureName></FeatureName></PrimaryAxis><SecondaryAxis><DefinedDirection>+X</DefinedDirection><Source>ReferenceFrame</Source><SourceDirection>+X</SourceDirection><FeatureName></FeatureName></SecondaryAxis></Value></Frame></Frames>  MarkerShape=Sphere  MarkerSize=10  GraphicType=FromGeometry  InertiaType=Custom  Mass=mParams.bodies.thigh.m  MassUnits=kg  MomentsOfInertia=mParams.bodies.thigh.In  MomentsOfInertiaUnits=kg*m^2  GraphicOpacity=1.0  ProductsOfInertia=[0 0 0]  ProductsOfInertiaUnits=kg*m^2  GraphicShininess=75  GraphicSpecularColor=[0.5 0.5 0.5 1.0]  GraphicVisPropType=SimpleVisualProperties
  Transform CG to MidSegment : sm_lib/Frames and Transforms/Rigid Transform  TranslationMethod=Cartesian  TranslationStandardOffset=0  TranslationLengthUnit=m  TranslationStandardAxis=+Y  TranslationCartesianOffset=[0 -mParams.bodies.thigh.l/2 0]  TranslationROffset=0  TranslationROffsetUnits=m  TranslationZOffset=0  TranslationZOffsetUnits=m  TranslationThetaOffset=0  TranslationThetaOffsetUnits=deg  RotationMethod=None  RotationAngleUnits=deg  RotationStandardAxis=+X  RotationAngle=90  RotationArbitraryAxis=[0 0 1]  FollAlignAxisA=+X  BaseAlignAxisA=+Y  FollAlignAxisB=+Y  BaseAlignAxisB=+Z  RotationSequenceAxes=FollowerAxes  RotationSequence=XYX  RotationSequenceAngles=[0 0 0]  RotationSequenceAnglesUnits=deg  RotationMatrix=[1 0 0; 0 1 0; 0 0 1]
  Transform CS1 to MidSegment : sm_lib/Frames and Transforms/Rigid Transform  TranslationMethod=Cartesian  TranslationStandardOffset=0  TranslationLengthUnit=m  TranslationStandardAxis=+Y  TranslationCartesianOffset=[0 -mParams.bodies.thigh.l/2 0]  TranslationROffset=0  TranslationROffsetUnits=m  TranslationZOffset=0  TranslationZOffsetUnits=m  TranslationThetaOffset=0  TranslationThetaOffsetUnits=deg  RotationMethod=None  RotationAngleUnits=deg  RotationStandardAxis=+X  RotationAngle=-90  RotationArbitraryAxis=[0 0 1]  FollAlignAxisA=+X  BaseAlignAxisA=+Y  FollAlignAxisB=+Y  BaseAlignAxisB=+Z  RotationSequenceAxes=FollowerAxes  RotationSequence=XYX  RotationSequenceAngles=[0 0 0]  RotationSequenceAnglesUnits=deg  RotationMatrix=[1 0 0; 0 1 0; 0 0 1]
  CS1 : PMIOPort  Side=Left
  CS2 : PMIOPort  Port=2  Side=Right
  connections:
  Transform CG to MidSegment/LConn1 -- Solid1/RConn1 -- Transform CS1 to MidSegment/RConn1
  Transform CS1 to MidSegment/LConn1 -- CS1/RConn1
  Transform CG to MidSegment/RConn1 -- CS2/RConn1

== system nmsRR/Body and Contact Model/Vestibular System/  XYZ Sensor Left Hip ==
  note: Simplified IMU Model
  Frame Sensor : sm_lib/Frames and Transforms/Transform Sensor  MeasurementFrame=World  SenseAngle=off  SenseAxis=off  SenseAngle1=off  SenseAngle2=off  SenseAngle3=off  SenseQ=off  SenseR=off  SenseOmegaX=off  SenseOmegaY=off  SenseOmegaZ=off  SenseOmega1=off  SenseOmega2=off  SenseOmega3=off  SenseQDot=off  SenseRDot=off  SenseAlphaX=off  SenseAlphaY=off  SenseAlphaZ=off  SenseAlpha1=off  SenseAlpha2=off  SenseAlpha3=off  SenseQDDot=off  SenseRDDot=off  SenseX=on  SenseY=on  SenseZ=on  SenseRad=off  SenseAzim=off  SenseDist=off  SenseInc=off  SenseXDot=on  SenseYDot=on  SenseZDot=on  SenseRadDot=off  SenseAzimDot=off  SenseDistDot=off  SenseIncDot=off  SenseXDDot=off  SenseYDDot=off  SenseZDDot=off  SenseRadDDot=off  SenseAzimDDot=off  SenseDistDDot=off  SenseIncDDot=off
  Mux1 : Mux  Inputs=3
  Mux3 : Mux  Inputs=3
  PS-Simulink Converter : nesl_utility/PS-Simulink Converter  PhysicalDomain=network_engine_domain  SubClassName=ps_output  LeftPortType=input  RightPortType=output  PseudoPeriodic=off  Frequencies=[]  Unit=m  AffineConversion=off
      settings: SourceProductBaseCode=PW,SS
  PS-Simulink Converter1 : nesl_utility/PS-Simulink Converter  PhysicalDomain=network_engine_domain  SubClassName=ps_output  LeftPortType=input  RightPortType=output  PseudoPeriodic=off  Frequencies=[]  Unit=m  AffineConversion=off
      settings: SourceProductBaseCode=PW,SS
  PS-Simulink Converter2 : nesl_utility/PS-Simulink Converter  PhysicalDomain=network_engine_domain  SubClassName=ps_output  LeftPortType=input  RightPortType=output  PseudoPeriodic=off  Frequencies=[]  Unit=m/s  AffineConversion=off
      settings: SourceProductBaseCode=PW,SS
  PS-Simulink Converter3 : nesl_utility/PS-Simulink Converter  PhysicalDomain=network_engine_domain  SubClassName=ps_output  LeftPortType=input  RightPortType=output  PseudoPeriodic=off  Frequencies=[]  Unit=m/s  AffineConversion=off
      settings: SourceProductBaseCode=PW,SS
  PS-Simulink Converter4 : nesl_utility/PS-Simulink Converter  PhysicalDomain=network_engine_domain  SubClassName=ps_output  LeftPortType=input  RightPortType=output  PseudoPeriodic=off  Frequencies=[]  Unit=m  AffineConversion=off
      settings: SourceProductBaseCode=PW,SS
  PS-Simulink Converter5 : nesl_utility/PS-Simulink Converter  PhysicalDomain=network_engine_domain  SubClassName=ps_output  LeftPortType=input  RightPortType=output  PseudoPeriodic=off  Frequencies=[]  Unit=m/s  AffineConversion=off
      settings: SourceProductBaseCode=PW,SS
  World Frame : sm_lib/Frames and Transforms/World Frame
  frame : PMIOPort  Side=Left
  Hip Position [m] : Outport  VectorParamsAs1DForOutWhenUnconnected=off
  Hip Velocity [m/s] : Outport  Port=2  VectorParamsAs1DForOutWhenUnconnected=off
  wires:
  PS-Simulink Converter4/1 -> Mux3/3
  PS-Simulink Converter/1 -> Mux3/1
  Mux3/1 -> Hip Position [m]/1
  PS-Simulink Converter1/1 -> Mux3/2
  PS-Simulink Converter3/1 -> Mux1/2
  PS-Simulink Converter5/1 -> Mux1/3
  PS-Simulink Converter2/1 -> Mux1/1
  Mux1/1 -> Hip Velocity [m/s]/1
  connections:
  Frame Sensor/RConn1 -- frame/RConn1
  World Frame/RConn1 -- Frame Sensor/LConn1
  Frame Sensor/RConn4 -- PS-Simulink Converter4/LConn1
  Frame Sensor/RConn3 -- PS-Simulink Converter1/LConn1
  Frame Sensor/RConn2 -- PS-Simulink Converter/LConn1
  Frame Sensor/RConn5 -- PS-Simulink Converter2/LConn1
  Frame Sensor/RConn6 -- PS-Simulink Converter3/LConn1
  Frame Sensor/RConn7 -- PS-Simulink Converter5/LConn1

== system nmsRR/Body and Contact Model/Vestibular System/  XYZ Sensor Right Hip ==
  note: Simplified IMU Model
  Frame Sensor : sm_lib/Frames and Transforms/Transform Sensor  MeasurementFrame=World  SenseAngle=off  SenseAxis=off  SenseAngle1=off  SenseAngle2=off  SenseAngle3=off  SenseQ=off  SenseR=off  SenseOmegaX=off  SenseOmegaY=off  SenseOmegaZ=off  SenseOmega1=off  SenseOmega2=off  SenseOmega3=off  SenseQDot=off  SenseRDot=off  SenseAlphaX=off  SenseAlphaY=off  SenseAlphaZ=off  SenseAlpha1=off  SenseAlpha2=off  SenseAlpha3=off  SenseQDDot=off  SenseRDDot=off  SenseX=on  SenseY=on  SenseZ=on  SenseRad=off  SenseAzim=off  SenseDist=off  SenseInc=off  SenseXDot=on  SenseYDot=on  SenseZDot=on  SenseRadDot=off  SenseAzimDot=off  SenseDistDot=off  SenseIncDot=off  SenseXDDot=off  SenseYDDot=off  SenseZDDot=off  SenseRadDDot=off  SenseAzimDDot=off  SenseDistDDot=off  SenseIncDDot=off
  Mux1 : Mux  Inputs=3
  Mux3 : Mux  Inputs=3
  PS-Simulink Converter : nesl_utility/PS-Simulink Converter  PhysicalDomain=network_engine_domain  SubClassName=ps_output  LeftPortType=input  RightPortType=output  PseudoPeriodic=off  Frequencies=[]  Unit=m  AffineConversion=off
      settings: SourceProductBaseCode=PW,SS
  PS-Simulink Converter1 : nesl_utility/PS-Simulink Converter  PhysicalDomain=network_engine_domain  SubClassName=ps_output  LeftPortType=input  RightPortType=output  PseudoPeriodic=off  Frequencies=[]  Unit=m  AffineConversion=off
      settings: SourceProductBaseCode=PW,SS
  PS-Simulink Converter2 : nesl_utility/PS-Simulink Converter  PhysicalDomain=network_engine_domain  SubClassName=ps_output  LeftPortType=input  RightPortType=output  PseudoPeriodic=off  Frequencies=[]  Unit=m/s  AffineConversion=off
      settings: SourceProductBaseCode=PW,SS
  PS-Simulink Converter3 : nesl_utility/PS-Simulink Converter  PhysicalDomain=network_engine_domain  SubClassName=ps_output  LeftPortType=input  RightPortType=output  PseudoPeriodic=off  Frequencies=[]  Unit=m/s  AffineConversion=off
      settings: SourceProductBaseCode=PW,SS
  PS-Simulink Converter4 : nesl_utility/PS-Simulink Converter  PhysicalDomain=network_engine_domain  SubClassName=ps_output  LeftPortType=input  RightPortType=output  PseudoPeriodic=off  Frequencies=[]  Unit=m  AffineConversion=off
      settings: SourceProductBaseCode=PW,SS
  PS-Simulink Converter5 : nesl_utility/PS-Simulink Converter  PhysicalDomain=network_engine_domain  SubClassName=ps_output  LeftPortType=input  RightPortType=output  PseudoPeriodic=off  Frequencies=[]  Unit=m/s  AffineConversion=off
      settings: SourceProductBaseCode=PW,SS
  World Frame : sm_lib/Frames and Transforms/World Frame
  frame : PMIOPort  Side=Left
  Hip Position [m] : Outport  VectorParamsAs1DForOutWhenUnconnected=off
  Hip Velocity [m/s] : Outport  Port=2  VectorParamsAs1DForOutWhenUnconnected=off
  wires:
  PS-Simulink Converter4/1 -> Mux3/3
  PS-Simulink Converter/1 -> Mux3/1
  Mux3/1 -> Hip Position [m]/1
  PS-Simulink Converter1/1 -> Mux3/2
  PS-Simulink Converter3/1 -> Mux1/2
  PS-Simulink Converter5/1 -> Mux1/3
  PS-Simulink Converter2/1 -> Mux1/1
  Mux1/1 -> Hip Velocity [m/s]/1
  connections:
  Frame Sensor/RConn1 -- frame/RConn1
  World Frame/RConn1 -- Frame Sensor/LConn1
  Frame Sensor/RConn4 -- PS-Simulink Converter4/LConn1
  Frame Sensor/RConn3 -- PS-Simulink Converter1/LConn1
  Frame Sensor/RConn2 -- PS-Simulink Converter/LConn1
  Frame Sensor/RConn5 -- PS-Simulink Converter2/LConn1
  Frame Sensor/RConn6 -- PS-Simulink Converter3/LConn1
  Frame Sensor/RConn7 -- PS-Simulink Converter5/LConn1

== system nmsRR/Body and Contact Model/Vestibular System/Align Axis ==
  note: Axis Alignment: We rotate the position vectors in the frame of the moving direction (R). For the lateral rotation, we measure the rotation of line that connects the two hip positions in the (0,0,1)-axis. For the saggital rotation, we measure the rotation of the line between Trunk-CoM (x,y,0) and the average position of the two hip joints (Hr+Hl)/2 in the (0,1,0)-axis
  Ankle Position Right [m] : Inport
  Ankle Position Left [m] : Inport  Port=2
  "R " : Inport  Port=3
  Position Trunk [m] : Inport  Port=4
  Velocity Trunk [m/s] : Inport  Port=5
  Hip Position Left [m] : Inport  Port=6
  Hip Position Right [m] : Inport  Port=7
  Compute Lateral Rotation : Subsystem
  Compute Saggital Rotation : Subsystem
  Matrix Multiply{,1..2,6..8} (6 alike) : Product  Multiplication=Matrix(*)
  Minus15 : Sum  Inputs=+-
  Minus2 : Sum  Inputs=+-
  Transfer Fcn (with initial outputs) : simulink_extras/Additional Linear/Transfer Fcn (with initial outputs)  N=[1 0]  D="[0.015  1]"  Y0=0  U0=0
  Transfer Fcn (with initial outputs)1 : simulink_extras/Additional Linear/Transfer Fcn (with initial outputs)  N=[1 0]  D="[0.015  1]"  Y0=0  U0=0
  Ankle Position Left (body frame) : Outport
  Ankle Position Right (body frame) : Outport  Port=2
  Trunk Velocity (body frame) : Outport  Port=3
  Saggital Trunk Rotation [rad] (body frame) : Outport  Port=4
  Lateral Trunk Rotation [rad] (body frame) : Outport  Port=5
  Saggital Trunk Rotation Velocity [rad/s] (body frame) : Outport  Port=6
  Lateral Trunk Rotation Velocity [rad/s] (body frame) : Outport  Port=7
  wires:
  Minus15/1 -> Matrix Multiply1/2
  Ankle Position Left [m]/1 -> Minus2/2
  Ankle Position Right [m]/1 -> Minus15/2
  Matrix Multiply/1 -> Ankle Position Left (body frame)/1
  Position Trunk [m]/1 -> Minus15/1, Matrix Multiply8/2, Minus2/1
  "R "/1 -> Matrix Multiply8/1, Matrix Multiply6/1, Matrix Multiply7/1, Matrix Multiply2/1, Matrix Multiply1/1, Matrix Multiply/1
  Minus2/1 -> Matrix Multiply/2
  Matrix Multiply1/1 -> Ankle Position Right (body frame)/1
  Velocity Trunk [m/s]/1 -> Matrix Multiply2/2
  Matrix Multiply2/1 -> Trunk Velocity (body frame)/1
  Hip Position Right [m]/1 -> Matrix Multiply6/2
  Hip Position Left [m]/1 -> Matrix Multiply7/2
  Compute Lateral Rotation/1(Lateral Rotation) -> Lateral Trunk Rotation [rad] (body frame)/1, Transfer Fcn (with initial outputs)/1
  Matrix Multiply7/1 -> Compute Saggital Rotation/1(Hip Position Left [m]), Compute Lateral Rotation/1(Hip Left)
  Matrix Multiply6/1 -> Compute Saggital Rotation/2(Hip Position Right [m]), Compute Lateral Rotation/2(Hip Right)
  Compute Saggital Rotation/1(Saggital Rotation) -> Saggital Trunk Rotation [rad] (body frame)/1, Transfer Fcn (with initial outputs)1/1
  Matrix Multiply8/1 -> Compute Saggital Rotation/3(Trunk Position [m])
  Transfer Fcn (with initial outputs)/1 -> Lateral Trunk Rotation Velocity [rad/s] (body frame)/1
  Transfer Fcn (with initial outputs)1/1 -> Saggital Trunk Rotation Velocity [rad/s] (body frame)/1

== system nmsRR/Body and Contact Model/Vestibular System/R Movement direction ==
  Hip Right : Inport
  Hip Left : Inport  Port=2
  Constant : Constant  Value=[0;1;0]
  Cross Product : vrlib/Utilities/Cross Product
  Gain : Gain  Gain=[1 0 1]
  Gain1 : Gain  Gain=[1 0 1]
  Matrix Concatenate : Concatenate  NumInputs=3  Mode=Multidimensional array  ConcatenateDimension=2
  Minus : Sum  Inputs=+-
  Transpose : Math  Operator=transpose  SaturateOnIntegerOverflow=on
  normalize : Subsystem
  "R " : Outport
  wires:
  Constant/1 -> Matrix Concatenate/2, Cross Product/1
  Hip Right/1 -> Gain/1
  Hip Left/1 -> Gain1/1
  Minus/1 -> normalize/1(vector)
  Matrix Concatenate/1 -> Transpose/1
  Transpose/1 -> "R "/1
  Cross Product/1 -> Matrix Concatenate/1
  Gain/1 -> Minus/1
  Gain1/1 -> Minus/2
  normalize/1(norm) -> Matrix Concatenate/3, Cross Product/2
